simulink model "sim_WAM_PBMCDynamics"  (R2018b)
settings: Solver=VariableStepAuto  StartTime=0.0  StopTime=10.0  FixedStep=1e-3  RelTol=1e-6
values from neighbouring files (symbols this model uses):
  Cfcn = handles.Cfcn    [GUI_WAM.m]    (also in convertSymVarsTOfunctions.m = matlabFunction(Ctemp, 'vars', {q1, q2, q4, q1d, q2d, q4d}))
  Ffcn = handles.Ffcn    [GUI_WAM.m]    (also in convertSymVarsTOfunctions.m = matlabFunction(Ftemp, 'vars', {q1d, q2d, q4d}))
  Gfcn = handles.Gfcn    [GUI_WAM.m]    (also in convertSymVarsTOfunctions.m = matlabFunction(Gtemp, 'vars', {q1, q2, q4}))
  handles =     [opt.mat]
  Mfcn = handles.Mfcn    [GUI_WAM.m]    (also in convertSymVarsTOfunctions.m = matlabFunction(Mtemp, 'vars', {q1, q2, q4}))
  TH = handles.TH    [GUI_WAM.m]    (also in THopt.m = [TH;X(41:46)]; WAM124YthetaRev.m = eval(TH); getWAMParameters.m = eval(TH))
  w = handles.w    [GUI_WAM.m]    (also in GetOptimalTrajectories.m = 0.628318530718; MAIN_FINAL.m = 1; MAIN_OptimalTrajectories.m = 0.628318530718; invDynWAM.m = 4)
  Yavfcn = handles.Yavfcn    [GUI_WAM.m]    (also in convertSymVarsTOfunctions.m = matlabFunction(Yavtemp, 'vars', {q1, q2, q4, q1d, q2d, q4d, )
undefined symbols (not defined in the file or in its folder): PBMC_WAM, statederWAM
settings Model: Creator=Erivelton  LastModifiedBy=Erivelton

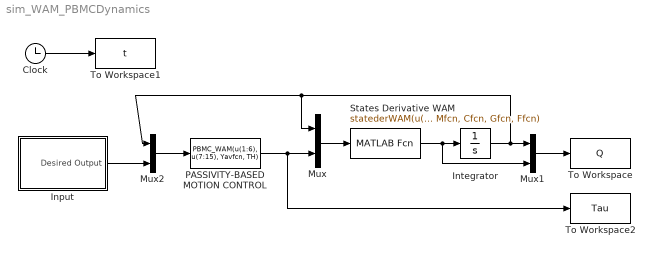
== system sim_WAM_PBMCDynamics ==
  Clock : Clock
  Input : Subsystem
  Integrator : Integrator  InitialCondition=handles.Q0
  Mux : Mux  Inputs=2
  Mux1 : Mux  Inputs=2
  Mux2 : Mux  Inputs=2
  PASSIVITY-BASED MOTION CONTROL : MATLABFcn  MATLABFcn=PBMC_WAM(u(1:6), u(7:15), Yavfcn, TH)  OutputDimensions=3
  States Derivative WAM : MATLABFcn  MATLABFcn=statederWAM(u(1:6), u(7:9), Mfcn, Cfcn, Gfcn, Ffcn)  OutputDimensions=6
  To Workspace : ToWorkspace  VariableName=Q  SampleTime=-1
  To Workspace1 : ToWorkspace  VariableName=t  SampleTime=-1
  To Workspace2 : ToWorkspace  VariableName=Tau  SampleTime=-1
  wires:
  States Derivative WAM/1 -> Mux1/2, Integrator/1
  Mux/1 -> States Derivative WAM/1
  Integrator/1 -> Mux1/1, Mux/1, Mux2/1
  Clock/1 -> To Workspace1/1
  Mux1/1 -> To Workspace/1
  Input/1(Desired Output) -> Mux2/2
  Mux2/1 -> PASSIVITY-BASED MOTION CONTROL/1
  PASSIVITY-BASED MOTION CONTROL/1 -> To Workspace2/1, Mux/2

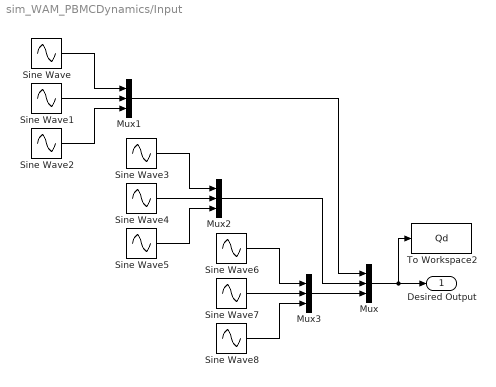
== system sim_WAM_PBMCDynamics/Input ==
  Mux{,1..3} (4 alike) : Mux  Inputs=3
  Sine Wave : Sin  Frequency=w  SampleTime=0
  Sine Wave1 : Sin  Amplitude=w  Frequency=w  Phase=pi/2  SampleTime=0
  Sine Wave2 : Sin  Amplitude=-w*w  Frequency=w  SampleTime=0
  Sine Wave3 : Sin  Bias=-.5  Frequency=w  SampleTime=0
  Sine Wave4 : Sin  Amplitude=w  Frequency=w  Phase=pi/2  SampleTime=0
  Sine Wave5 : Sin  Amplitude=-w*w  Frequency=w  SampleTime=0
  Sine Wave6 : Sin  Amplitude=.75  Frequency=w  SampleTime=0
  Sine Wave7 : Sin  Amplitude=.75*w  Frequency=w  Phase=pi/2  SampleTime=0
  Sine Wave8 : Sin  Amplitude=-.75*w*w  Frequency=w  SampleTime=0
  To Workspace2 : ToWorkspace  VariableName=Qd  SampleTime=-1
  Desired Output : Outport
  wires:
  Mux/1 -> To Workspace2/1, Desired Output/1
  Mux3/1 -> Mux/3
  Mux2/1 -> Mux/2
  Mux1/1 -> Mux/1
  Sine Wave/1 -> Mux1/1
  Sine Wave1/1 -> Mux1/2
  Sine Wave2/1 -> Mux1/3
  Sine Wave5/1 -> Mux2/3
  Sine Wave4/1 -> Mux2/2
  Sine Wave3/1 -> Mux2/1
  Sine Wave8/1 -> Mux3/3
  Sine Wave7/1 -> Mux3/2
  Sine Wave6/1 -> Mux3/1
